simulink model "sampleModel56"  (Simulink 9.1)
settings: Solver=VariableStepAuto  StartTime=0.0  StopTime=10.0  RelTol=1e-3
undefined symbols (not defined in the file): DiscIntNeverNeededParam, Newton, Raphson
libraries: simulink x48
(part 2 of 2)

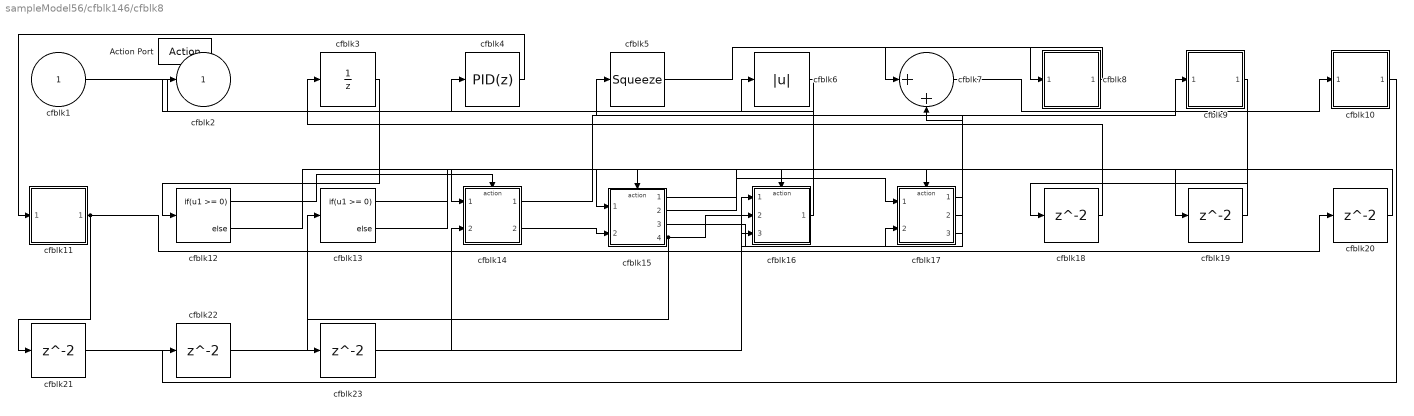
== system sampleModel56/cfblk146/cfblk8 ==
  cfblk1 : Inport
  Action Port : ActionPort  ActionType=then
  cfblk10 : Subsystem
  cfblk11 : Subsystem
  cfblk12 : If  IfExpression=u1 >= 0  SampleTime=1
  cfblk13 : If  IfExpression=u1 >= 0  SampleTime=1
  cfblk14 : Subsystem  TreatAsAtomicUnit=on
  cfblk15 : Subsystem  TreatAsAtomicUnit=on
  cfblk16 : Subsystem  TreatAsAtomicUnit=on
  cfblk17 : Subsystem  TreatAsAtomicUnit=on
  cfblk{18..23} (6 alike) : Delay
  cfblk3 : UnitDelay  SampleTime=-1
  cfblk4 : simulink/Continuous/PID Controller  Controller=PID  TimeDomain=Discrete-time  SampleTime=-1  IntegratorMethod=Forward Euler  FilterMethod=Forward Euler  Form=Parallel  UseFilter=on  ControllerParametersSource=internal  P=1  I=1  D=0  N=100  InitialConditionSource=internal  InitialConditionForIntegrator=0  InitialConditionForFilter=0  ExternalReset=none  LimitOutput=off  UpperSaturationLimit=inf  LowerSaturationLimit=-inf  LinearizeAsGain=off  AntiWindupMode=none  Kb=1  TrackingMode=off  Kt=1  PParamMin=[]  PParamMax=[]  IParamMin=[]  IParamMax=[]  DParamMin=[]  DParamMax=[]  NParamMin=[]  NParamMax=[]  KbParamMin=[]  KbParamMax=[]  KtParamMin=[]  KtParamMax=[]  POutMin=[]  POutMax=[]  IOutMin=[]  IOutMax=[]  DOutMin=[]  DOutMax=[]  NOutMin=[]  NOutMax=[]  KbOutMin=[]  KbOutMax=[]  KtOutMin=[]  KtOutMax=[]  IntegratorOutMin=[]  IntegratorOutMax=[]  FilterOutMin=[]  FilterOutMax=[]  SumOutMin=[]  SumOutMax=[]  SumI1OutMin=[]  SumI1OutMax=[]  SumI2OutMin=[]  SumI2OutMax=[]  SumI3OutMin=[]  SumI3OutMax=[]  SumDOutMin=[]  SumDOutMax=[]  SaturationOutMin=[]  SaturationOutMax=[]  IntegratorContinuousStateAttributes=''  IntegratorStateMustResolveToSignalObject=off  IntegratorRTWStateStorageClass=Auto  FilterContinuousStateAttributes=''  FilterStateMustResolveToSignalObject=off  FilterRTWStateStorageClass=Auto  DifferentiatorICPrevScaledInput=0  DifferentiatorOutMin=[]  DifferentiatorOutMax=[]  FilterDiffOutCoefMin=[]  FilterDiffOutCoefMax=[]  SumDenOutMin=[]  SumDenOutMax=[]  SumNumOutMin=[]  SumNumOutMax=[]  ReciprocalOutMin=[]  ReciprocalOutMax=[]  DivideOutMin=[]  DivideOutMax=[]  TunerSelectOption=Transfer Function Based (PID Tuner App)
  cfblk5 : Squeeze
  cfblk6 : Abs
  cfblk7 : Sum  Inputs=|++
  cfblk8 : Subsystem
  cfblk9 : Subsystem
  cfblk2 : Outport
  wires:
  cfblk1/1 -> cfblk6/1
  cfblk3/1 -> cfblk12/1
  cfblk4/1 -> cfblk11/1(cfblk1)
  cfblk6/1 -> cfblk2/1
  cfblk5/1 -> cfblk8/1(cfblk1)
  cfblk16/1(cfblk2) -> cfblk4/1
  cfblk11/1(cfblk2) -> cfblk20/1, cfblk21/1
  cfblk7/1 -> cfblk10/1(cfblk1)
  cfblk14/1(cfblk2) -> cfblk9/1(cfblk1)
  cfblk8/1(cfblk2) -> cfblk7/1
  cfblk14/2(cfblk12) -> cfblk15/2(cfblk12)
  cfblk17/1(cfblk2) -> cfblk16/1(cfblk1)
  cfblk17/2(cfblk16) -> cfblk5/1
  cfblk17/3(cfblk17) -> cfblk7/2
  cfblk15/2(cfblk13) -> cfblk17/1(cfblk1)
  cfblk15/3(cfblk14) -> cfblk17/2(cfblk15)
  cfblk15/4(cfblk15) -> cfblk16/2(cfblk15), cfblk23/1
  cfblk12/1 -> cfblk14/Action
  cfblk12/2 -> cfblk15/Action
  cfblk13/1 -> cfblk16/Action
  cfblk13/2 -> cfblk17/Action
  cfblk9/1(cfblk2) -> cfblk18/1
  cfblk18/1 -> cfblk3/1
  cfblk15/1(cfblk2) -> cfblk19/1
  cfblk19/1 -> cfblk14/1(cfblk1)
  cfblk20/1 -> cfblk15/1(cfblk1)
  cfblk21/1 -> cfblk16/3(cfblk16)
  cfblk10/1(cfblk2) -> cfblk22/1
  cfblk22/1 -> cfblk13/1
  cfblk23/1 -> cfblk14/2(cfblk11)

== system sampleModel56/cfblk146/cfblk9 ==
  cfblk1 : Inport
  Action Port : ActionPort  ActionType=else
  cfblk3 : UnitDelay  SampleTime=-1
  cfblk4 : Product  Inputs=*
  cfblk5 : Subsystem
  cfblk6 : Subsystem
  cfblk7 : Subsystem
  cfblk8 : Subsystem
  cfblk2 : Outport
  cfblk9 : Outport  Port=2
  wires:
  cfblk1/1 -> cfblk8/1(cfblk1)
  cfblk8/1(cfblk2) -> cfblk6/1(cfblk1)
  cfblk6/1(cfblk2) -> cfblk7/1(cfblk1)
  cfblk7/1(cfblk2) -> cfblk3/1, cfblk5/1(cfblk1)
  cfblk3/1 -> cfblk2/1
  cfblk5/1(cfblk2) -> cfblk4/1
  cfblk4/1 -> cfblk9/1

== system sampleModel56/cfblk147/cfblk10 ==
  cfblk1 : Inport
  cfblk2 : Outport
  wires:
  cfblk1/1 -> cfblk2/1

== system sampleModel56/cfblk147/cfblk11 ==
  cfblk1 : Inport
  cfblk2 : Outport
  wires:
  cfblk1/1 -> cfblk2/1

== system sampleModel56/cfblk147/cfblk12 ==
  cfblk1 : Inport
  cfblk2 : Outport
  wires:
  cfblk1/1 -> cfblk2/1

== system sampleModel56/cfblk147/cfblk13 ==
  cfblk1 : Inport
  cfblk2 : Outport
  wires:
  cfblk1/1 -> cfblk2/1

== system sampleModel56/cfblk147/cfblk14 ==
  cfblk1 : Inport
  cfblk2 : Outport
  wires:
  cfblk1/1 -> cfblk2/1

== system sampleModel56/cfblk148/cfblk10 ==
  cfblk1 : Inport
  cfblk2 : Outport
  wires:
  cfblk1/1 -> cfblk2/1

== system sampleModel56/cfblk148/cfblk11 ==
  cfblk1 : Inport
  cfblk2 : Outport
  wires:
  cfblk1/1 -> cfblk2/1

== system sampleModel56/cfblk148/cfblk12 ==
  cfblk1 : Inport
  cfblk2 : Outport
  wires:
  cfblk1/1 -> cfblk2/1

== system sampleModel56/cfblk148/cfblk13 ==
  cfblk1 : Inport
  cfblk2 : Outport
  wires:
  cfblk1/1 -> cfblk2/1

== system sampleModel56/cfblk148/cfblk9 ==
  cfblk1 : Inport
  cfblk2 : Outport
  wires:
  cfblk1/1 -> cfblk2/1

== system sampleModel56/cfblk149/cfblk10 ==
  cfblk1 : Inport
  cfblk2 : Outport
  wires:
  cfblk1/1 -> cfblk2/1

== system sampleModel56/cfblk149/cfblk11 ==
  cfblk1 : Inport
  cfblk2 : Outport
  wires:
  cfblk1/1 -> cfblk2/1

== system sampleModel56/cfblk149/cfblk9 ==
  cfblk1 : Inport
  cfblk2 : Outport
  wires:
  cfblk1/1 -> cfblk2/1

== system sampleModel56/cfblk150/cfblk6 ==
  cfblk1 : Inport
  cfblk2 : Outport
  wires:
  cfblk1/1 -> cfblk2/1

== system sampleModel56/cfblk150/cfblk7 ==
  cfblk1 : Inport
  cfblk2 : Outport
  wires:
  cfblk1/1 -> cfblk2/1

== system sampleModel56/cfblk152/cfblk11 ==
  cfblk1 : Inport
  Action Port : ActionPort  ActionType=then
  cfblk10 : Subsystem
  cfblk11 : Subsystem
  cfblk3 : DiscreteTransferFcn
  cfblk4 : UnitDelay  SampleTime=-1
  cfblk5 : DiscreteIntegrator  SampleTime=-1  ICPrevOutput=DiscIntNeverNeededParam  ICPrevScaledInput=DiscIntNeverNeededParam
  cfblk6 : Sqrt  SaturateOnIntegerOverflow=on
  cfblk7 : Gain  Gain=[470576292.236771]
  cfblk8 : Subsystem
  cfblk9 : Subsystem
  cfblk2 : Outport
  cfblk12 : Outport  Port=2
  cfblk13 : Outport  Port=3
  wires:
  cfblk7/1 -> cfblk4/1
  cfblk6/1 -> cfblk7/1
  cfblk1/1 -> cfblk10/1(cfblk1)
  cfblk4/1 -> cfblk5/1
  cfblk11/1(cfblk2) -> cfblk8/1(cfblk1), cfblk2/1
  cfblk8/1(cfblk2) -> cfblk3/1
  cfblk3/1 -> cfblk12/1
  cfblk9/1(cfblk2) -> cfblk11/1(cfblk1)
  cfblk5/1 -> cfblk13/1, cfblk9/1(cfblk1)
  cfblk10/1(cfblk2) -> cfblk6/1

== system sampleModel56/cfblk152/cfblk12 ==
  cfblk1 : Inport
  cfblk9 : Inport  Port=2
  cfblk10 : Inport  Port=3
  Action Port : ActionPort  ActionType=else
  cfblk3 : UnitDelay  SampleTime=-1
  cfblk4 : Abs
  cfblk5 : Bias  Bias=[477951449.519788]
  cfblk6 : Signum
  cfblk7 : Subsystem
  cfblk8 : Subsystem
  cfblk2 : Outport
  wires:
  cfblk5/1 -> cfblk2/1
  cfblk6/1 -> cfblk4/1
  cfblk9/1 -> cfblk3/1
  cfblk4/1 -> cfblk8/1(cfblk1)
  cfblk10/1 -> cfblk5/1
  cfblk1/1 -> cfblk6/1
  cfblk8/1(cfblk2) -> cfblk7/1(cfblk1)

== system sampleModel56/cfblk152/cfblk6 ==
  cfblk1 : Inport
  cfblk2 : Outport
  wires:
  cfblk1/1 -> cfblk2/1

== system sampleModel56/cfblk152/cfblk7 ==
  cfblk1 : Inport
  cfblk2 : Outport
  wires:
  cfblk1/1 -> cfblk2/1

== system sampleModel56/cfblk152/cfblk8 ==
  cfblk1 : Inport
  cfblk2 : Outport
  wires:
  cfblk1/1 -> cfblk2/1

== system sampleModel56/cfblk153/cfblk11 ==
  cfblk1 : Inport
  cfblk2 : Outport
  wires:
  cfblk1/1 -> cfblk2/1

== system sampleModel56/cfblk153/cfblk12 ==
  cfblk1 : Inport
  cfblk2 : Outport
  wires:
  cfblk1/1 -> cfblk2/1

== system sampleModel56/cfblk154/cfblk11 ==
  cfblk1 : Inport
  cfblk2 : Outport
  wires:
  cfblk1/1 -> cfblk2/1

== system sampleModel56/cfblk154/cfblk12 ==
  cfblk1 : Inport
  cfblk2 : Outport
  wires:
  cfblk1/1 -> cfblk2/1

== system sampleModel56/cfblk154/cfblk13 ==
  cfblk1 : Inport
  cfblk2 : Outport
  wires:
  cfblk1/1 -> cfblk2/1

== system sampleModel56/cfblk154/cfblk14 ==
  cfblk1 : Inport
  cfblk2 : Outport
  wires:
  cfblk1/1 -> cfblk2/1

== system sampleModel56/cfblk155/cfblk10 ==
  cfblk1 : Inport
  cfblk2 : Outport
  wires:
  cfblk1/1 -> cfblk2/1

== system sampleModel56/cfblk155/cfblk7 ==
  cfblk1 : Inport
  cfblk2 : Outport
  wires:
  cfblk1/1 -> cfblk2/1

== system sampleModel56/cfblk155/cfblk8 ==
  cfblk1 : Inport
  cfblk2 : Outport
  wires:
  cfblk1/1 -> cfblk2/1

== system sampleModel56/cfblk155/cfblk9 ==
  cfblk1 : Inport
  cfblk2 : Outport
  wires:
  cfblk1/1 -> cfblk2/1

== system sampleModel56/cfblk156/cfblk10 ==
  cfblk1 : Inport
  cfblk2 : Outport
  wires:
  cfblk1/1 -> cfblk2/1

== system sampleModel56/cfblk156/cfblk11 ==
  cfblk1 : Inport
  cfblk2 : Outport
  wires:
  cfblk1/1 -> cfblk2/1

== system sampleModel56/cfblk156/cfblk12 ==
  cfblk1 : Inport
  cfblk2 : Outport
  wires:
  cfblk1/1 -> cfblk2/1

== system sampleModel56/cfblk156/cfblk9 ==
  cfblk1 : Inport
  cfblk2 : Outport
  wires:
  cfblk1/1 -> cfblk2/1

== system sampleModel56/cfblk157/cfblk7 ==
  cfblk1 : Inport
  cfblk2 : Outport
  wires:
  cfblk1/1 -> cfblk2/1

== system sampleModel56/cfblk157/cfblk8 ==
  cfblk1 : Inport
  cfblk2 : Outport
  wires:
  cfblk1/1 -> cfblk2/1

== system sampleModel56/cfblk158/cfblk10 ==
  cfblk1 : Inport
  cfblk2 : Outport
  wires:
  cfblk1/1 -> cfblk2/1

== system sampleModel56/cfblk158/cfblk11 ==
  cfblk1 : Inport
  cfblk2 : Outport
  wires:
  cfblk1/1 -> cfblk2/1

== system sampleModel56/cfblk158/cfblk12 ==
  cfblk1 : Inport
  cfblk2 : Outport
  wires:
  cfblk1/1 -> cfblk2/1

== system sampleModel56/cfblk158/cfblk13 ==
  cfblk1 : Inport
  cfblk2 : Outport
  wires:
  cfblk1/1 -> cfblk2/1

== system sampleModel56/cfblk158/cfblk14 ==
  cfblk1 : Inport
  cfblk2 : Outport
  wires:
  cfblk1/1 -> cfblk2/1

== system sampleModel56/cfblk158/cfblk15 ==
  cfblk1 : Inport
  cfblk2 : Outport
  wires:
  cfblk1/1 -> cfblk2/1

== system sampleModel56/cfblk158/cfblk8 ==
  cfblk1 : Inport
  cfblk2 : Outport
  wires:
  cfblk1/1 -> cfblk2/1

== system sampleModel56/cfblk158/cfblk9 ==
  cfblk1 : Inport
  cfblk2 : Outport
  wires:
  cfblk1/1 -> cfblk2/1

== system sampleModel56/cfblk146/cfblk8/cfblk10 ==
  cfblk1 : Inport
  cfblk2 : Outport
  wires:
  cfblk1/1 -> cfblk2/1

== system sampleModel56/cfblk146/cfblk8/cfblk11 ==
  cfblk1 : Inport
  cfblk2 : Outport
  wires:
  cfblk1/1 -> cfblk2/1

== system sampleModel56/cfblk146/cfblk8/cfblk14 ==
  cfblk1 : Inport
  cfblk11 : Inport  Port=2
  Action Port : ActionPort  ActionType=then
  cfblk10 : Subsystem
  cfblk13 : Delay
  cfblk14 : Delay
  cfblk3 : DiscreteTransferFcn
  cfblk4 : Delay  ShowEnablePort=on
      settings: InputPortMap=u0,e6
  cfblk5 : Sqrt  SaturateOnIntegerOverflow=on
  cfblk6 : Reshape
  cfblk7 : DotProduct  InputSameDT=on  OutDataTypeStr=Inherit: Inherit via internal rule
  cfblk8 : Product  Inputs=*
  cfblk9 : Subsystem
  cfblk2 : Outport
  cfblk12 : Outport  Port=2
  wires:
  cfblk4/1 -> cfblk9/1(cfblk1), cfblk7/2, cfblk6/1
  cfblk11/1 -> cfblk12/1
  cfblk3/1 -> cfblk10/1(cfblk1)
  cfblk6/1 -> cfblk5/1
  cfblk1/1 -> cfblk8/1
  cfblk5/1 -> cfblk7/1
  cfblk8/1 -> cfblk4/2
  cfblk7/1 -> cfblk2/1
  cfblk9/1(cfblk2) -> cfblk13/1
  cfblk13/1 -> cfblk4/1
  cfblk10/1(cfblk2) -> cfblk14/1
  cfblk14/1 -> cfblk3/1

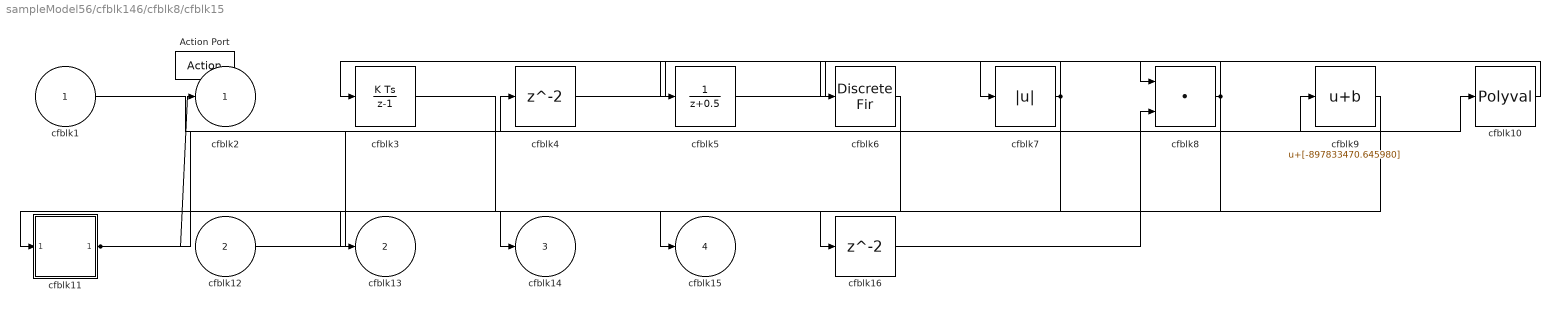
== system sampleModel56/cfblk146/cfblk8/cfblk15 ==
  cfblk1 : Inport
  cfblk12 : Inport  Port=2
  Action Port : ActionPort  ActionType=else
  cfblk10 : Polyval  Coefs=[ +2.081618890e-019, -1.441693666e-014, +4.719686976e-010, -8.536869453e-006, +1.621573104e-001, -8.087801117e+001 ]
  cfblk11 : Subsystem
  cfblk16 : Delay
  cfblk3 : DiscreteIntegrator  SampleTime=-1  ICPrevOutput=DiscIntNeverNeededParam  ICPrevScaledInput=DiscIntNeverNeededParam
  cfblk4 : Delay
  cfblk5 : DiscreteTransferFcn
  cfblk6 : DiscreteFir
  cfblk7 : Abs
  cfblk8 : DotProduct  InputSameDT=on  OutDataTypeStr=Inherit: Inherit via internal rule
  cfblk9 : Bias  Bias=[-897833470.645980]
  cfblk2 : Outport
  cfblk13 : Outport  Port=2
  cfblk14 : Outport  Port=3
  cfblk15 : Outport  Port=4
  wires:
  cfblk9/1 -> cfblk14/1
  cfblk12/1 -> cfblk9/1
  cfblk10/1 -> cfblk3/1
  cfblk4/1 -> cfblk8/1
  cfblk1/1 -> cfblk4/1
  cfblk6/1 -> cfblk15/1
  cfblk5/1 -> cfblk7/1
  cfblk7/1 -> cfblk6/1, cfblk13/1
  cfblk8/1 -> cfblk5/1, cfblk11/1(cfblk1)
  cfblk11/1(cfblk2) -> cfblk2/1, cfblk10/1
  cfblk3/1 -> cfblk16/1
  cfblk16/1 -> cfblk8/2

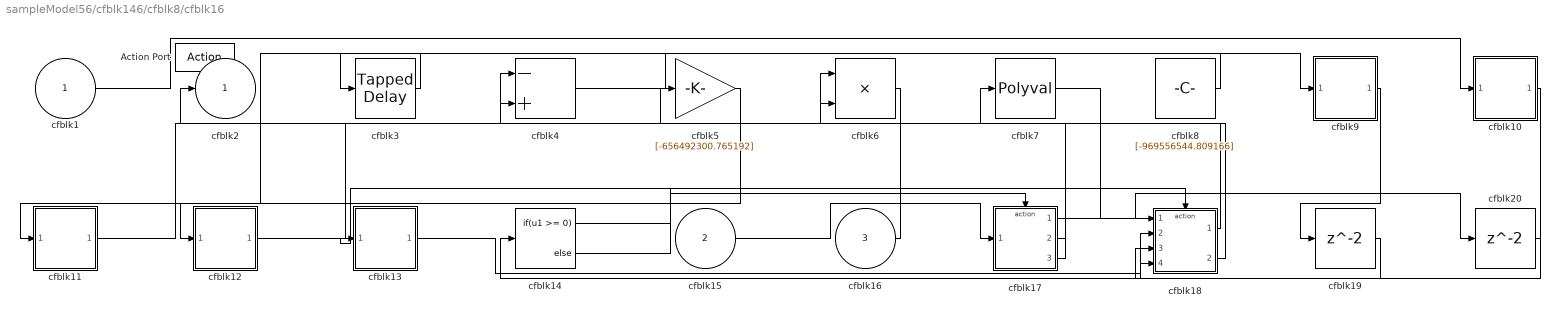
== system sampleModel56/cfblk146/cfblk8/cfblk16 ==
  cfblk1 : Inport
  cfblk15 : Inport  Port=2
  cfblk16 : Inport  Port=3
  Action Port : ActionPort  ActionType=then
  cfblk10 : Subsystem
  cfblk11 : Subsystem
  cfblk12 : Subsystem
  cfblk13 : Subsystem
  cfblk14 : If  IfExpression=u1 >= 0  SampleTime=1
  cfblk17 : Subsystem  TreatAsAtomicUnit=on
  cfblk18 : Subsystem  TreatAsAtomicUnit=on
  cfblk19 : Delay
  cfblk20 : Delay
  cfblk3 : simulink/Discrete/Tapped Delay  vinit=0.0  samptime=-1  NumDelays=1  DelayOrder=Oldest  includeCurrent=off
  cfblk4 : Sum  Inputs=-+
  cfblk5 : Gain  Gain=[-656492300.765192]
  cfblk6 : Product  Inputs=**
  cfblk7 : Polyval  Coefs=[ +2.081618890e-019, -1.441693666e-014, +4.719686976e-010, -8.536869453e-006, +1.621573104e-001, -8.087801117e+001 ]
  cfblk8 : Constant  Value=[-969556544.809166]  SampleTime=1
  cfblk9 : Subsystem
  cfblk2 : Outport
  wires:
  cfblk7/1 -> cfblk18/1(cfblk1)
  cfblk10/1(cfblk2) -> cfblk18/2(cfblk8)
  cfblk12/1(cfblk2) -> cfblk4/1
  cfblk6/1 -> cfblk13/1(cfblk1)
  cfblk3/1 -> cfblk12/1(cfblk1)
  cfblk15/1 -> cfblk17/1(cfblk1)
  cfblk8/1 -> cfblk3/1
  cfblk1/1 -> cfblk10/1(cfblk1)
  cfblk4/1 -> cfblk9/1(cfblk1)
  cfblk18/1(cfblk2) -> cfblk5/1
  cfblk16/1 -> cfblk6/1
  cfblk11/1(cfblk2) -> cfblk4/2
  cfblk17/2(cfblk12) -> cfblk6/2
  cfblk18/2(cfblk11) -> cfblk2/1
  cfblk13/1(cfblk2) -> cfblk18/4(cfblk10)
  cfblk17/3(cfblk13) -> cfblk7/1
  cfblk5/1 -> cfblk11/1(cfblk1)
  cfblk14/1 -> cfblk17/Action
  cfblk14/2 -> cfblk18/Action
  cfblk9/1(cfblk2) -> cfblk19/1
  cfblk19/1 -> cfblk18/3(cfblk9)
  cfblk17/1(cfblk2) -> cfblk20/1
  cfblk20/1 -> cfblk14/1

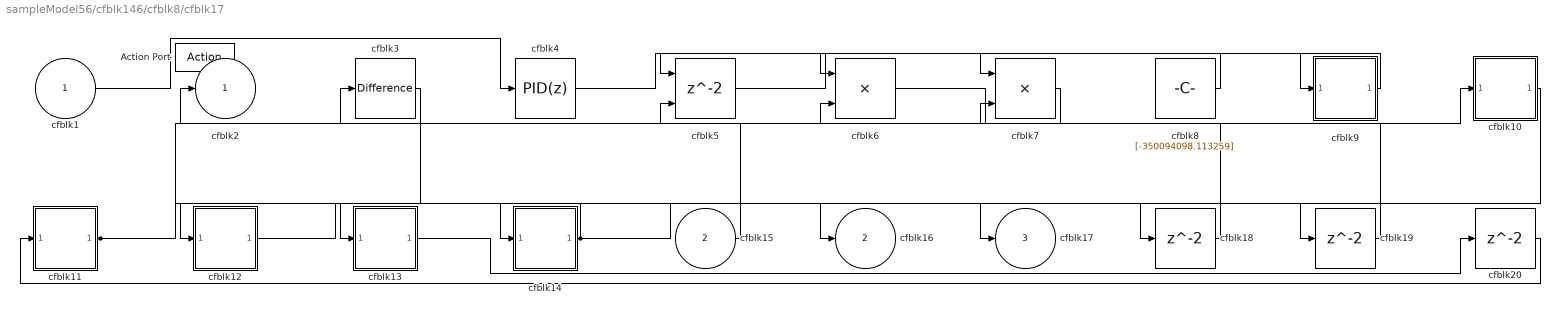
== system sampleModel56/cfblk146/cfblk8/cfblk17 ==
  cfblk1 : Inport
  cfblk15 : Inport  Port=2
  Action Port : ActionPort  ActionType=else
  cfblk10 : Subsystem
  cfblk11 : Subsystem
  cfblk12 : Subsystem
  cfblk13 : Subsystem
  cfblk14 : Subsystem
  cfblk18 : Delay
  cfblk19 : Delay
  cfblk20 : Delay
  cfblk3 : simulink/Discrete/Difference  ICPrevInput=0.0  OutMin=[]  OutMax=[]  OutDataTypeStr=Inherit: Inherit via back propagation  OutDataType=fixdt(1, 16)  OutScaling=2^-10  DoSatur=off
  cfblk4 : simulink/Continuous/PID Controller  Controller=PID  TimeDomain=Discrete-time  SampleTime=-1  IntegratorMethod=Forward Euler  FilterMethod=Forward Euler  Form=Parallel  UseFilter=on  ControllerParametersSource=internal  P=1  I=1  D=0  N=100  InitialConditionSource=internal  InitialConditionForIntegrator=0  InitialConditionForFilter=0  ExternalReset=none  LimitOutput=off  UpperSaturationLimit=inf  LowerSaturationLimit=-inf  LinearizeAsGain=off  AntiWindupMode=none  Kb=1  TrackingMode=off  Kt=1  PParamMin=[]  PParamMax=[]  IParamMin=[]  IParamMax=[]  DParamMin=[]  DParamMax=[]  NParamMin=[]  NParamMax=[]  KbParamMin=[]  KbParamMax=[]  KtParamMin=[]  KtParamMax=[]  POutMin=[]  POutMax=[]  IOutMin=[]  IOutMax=[]  DOutMin=[]  DOutMax=[]  NOutMin=[]  NOutMax=[]  KbOutMin=[]  KbOutMax=[]  KtOutMin=[]  KtOutMax=[]  IntegratorOutMin=[]  IntegratorOutMax=[]  FilterOutMin=[]  FilterOutMax=[]  SumOutMin=[]  SumOutMax=[]  SumI1OutMin=[]  SumI1OutMax=[]  SumI2OutMin=[]  SumI2OutMax=[]  SumI3OutMin=[]  SumI3OutMax=[]  SumDOutMin=[]  SumDOutMax=[]  SaturationOutMin=[]  SaturationOutMax=[]  IntegratorContinuousStateAttributes=''  IntegratorStateMustResolveToSignalObject=off  IntegratorRTWStateStorageClass=Auto  FilterContinuousStateAttributes=''  FilterStateMustResolveToSignalObject=off  FilterRTWStateStorageClass=Auto  DifferentiatorICPrevScaledInput=0  DifferentiatorOutMin=[]  DifferentiatorOutMax=[]  FilterDiffOutCoefMin=[]  FilterDiffOutCoefMax=[]  SumDenOutMin=[]  SumDenOutMax=[]  SumNumOutMin=[]  SumNumOutMax=[]  ReciprocalOutMin=[]  ReciprocalOutMax=[]  DivideOutMin=[]  DivideOutMax=[]  TunerSelectOption=Transfer Function Based (PID Tuner App)
  cfblk5 : Delay  ShowEnablePort=on
      settings: InputPortMap=u0,e6
  cfblk6 : Product  Inputs=**
  cfblk7 : Product
  cfblk8 : Constant  Value=[-350094098.113259]  SampleTime=1
  cfblk9 : Subsystem
  cfblk2 : Outport
  cfblk16 : Outport  Port=2
  cfblk17 : Outport  Port=3
  wires:
  cfblk15/1 -> cfblk2/1
  cfblk8/1 -> cfblk5/1
  cfblk3/1 -> cfblk12/1(cfblk1)
  cfblk7/1 -> cfblk5/2
  cfblk1/1 -> cfblk4/1
  cfblk5/1 -> cfblk9/1(cfblk1)
  cfblk14/1(cfblk2) -> cfblk13/1(cfblk1), cfblk17/1
  cfblk4/1 -> cfblk7/1
  cfblk6/1 -> cfblk10/1(cfblk1)
  cfblk11/1(cfblk2) -> cfblk7/2, cfblk16/1, cfblk14/1(cfblk1)
  cfblk9/1(cfblk2) -> cfblk6/1
  cfblk10/1(cfblk2) -> cfblk18/1
  cfblk18/1 -> cfblk6/2
  cfblk12/1(cfblk2) -> cfblk19/1
  cfblk19/1 -> cfblk3/1
  cfblk13/1(cfblk2) -> cfblk20/1
  cfblk20/1 -> cfblk11/1(cfblk1)

== system sampleModel56/cfblk146/cfblk8/cfblk8 ==
  cfblk1 : Inport
  cfblk2 : Outport
  wires:
  cfblk1/1 -> cfblk2/1

== system sampleModel56/cfblk146/cfblk8/cfblk9 ==
  cfblk1 : Inport
  cfblk2 : Outport
  wires:
  cfblk1/1 -> cfblk2/1

== system sampleModel56/cfblk146/cfblk9/cfblk5 ==
  cfblk1 : Inport
  cfblk2 : Outport
  wires:
  cfblk1/1 -> cfblk2/1

== system sampleModel56/cfblk146/cfblk9/cfblk6 ==
  cfblk1 : Inport
  cfblk2 : Outport
  wires:
  cfblk1/1 -> cfblk2/1

== system sampleModel56/cfblk146/cfblk9/cfblk7 ==
  cfblk1 : Inport
  cfblk2 : Outport
  wires:
  cfblk1/1 -> cfblk2/1

== system sampleModel56/cfblk146/cfblk9/cfblk8 ==
  cfblk1 : Inport
  cfblk2 : Outport
  wires:
  cfblk1/1 -> cfblk2/1

== system sampleModel56/cfblk152/cfblk11/cfblk10 ==
  cfblk1 : Inport
  cfblk2 : Outport
  wires:
  cfblk1/1 -> cfblk2/1

== system sampleModel56/cfblk152/cfblk11/cfblk11 ==
  cfblk1 : Inport
  cfblk2 : Outport
  wires:
  cfblk1/1 -> cfblk2/1

== system sampleModel56/cfblk152/cfblk11/cfblk8 ==
  cfblk1 : Inport
  cfblk2 : Outport
  wires:
  cfblk1/1 -> cfblk2/1

== system sampleModel56/cfblk152/cfblk11/cfblk9 ==
  cfblk1 : Inport
  cfblk2 : Outport
  wires:
  cfblk1/1 -> cfblk2/1

== system sampleModel56/cfblk152/cfblk12/cfblk7 ==
  cfblk1 : Inport
  cfblk2 : Outport
  wires:
  cfblk1/1 -> cfblk2/1

== system sampleModel56/cfblk152/cfblk12/cfblk8 ==
  cfblk1 : Inport
  cfblk2 : Outport
  wires:
  cfblk1/1 -> cfblk2/1

== system sampleModel56/cfblk146/cfblk8/cfblk14/cfblk10 ==
  cfblk1 : Inport
  cfblk2 : Outport
  wires:
  cfblk1/1 -> cfblk2/1

== system sampleModel56/cfblk146/cfblk8/cfblk14/cfblk9 ==
  cfblk1 : Inport
  cfblk2 : Outport
  wires:
  cfblk1/1 -> cfblk2/1

== system sampleModel56/cfblk146/cfblk8/cfblk15/cfblk11 ==
  cfblk1 : Inport
  cfblk2 : Outport
  wires:
  cfblk1/1 -> cfblk2/1

== system sampleModel56/cfblk146/cfblk8/cfblk16/cfblk10 ==
  cfblk1 : Inport
  cfblk2 : Outport
  wires:
  cfblk1/1 -> cfblk2/1

== system sampleModel56/cfblk146/cfblk8/cfblk16/cfblk11 ==
  cfblk1 : Inport
  cfblk2 : Outport
  wires:
  cfblk1/1 -> cfblk2/1

== system sampleModel56/cfblk146/cfblk8/cfblk16/cfblk12 ==
  cfblk1 : Inport
  cfblk2 : Outport
  wires:
  cfblk1/1 -> cfblk2/1

== system sampleModel56/cfblk146/cfblk8/cfblk16/cfblk13 ==
  cfblk1 : Inport
  cfblk2 : Outport
  wires:
  cfblk1/1 -> cfblk2/1

== system sampleModel56/cfblk146/cfblk8/cfblk16/cfblk17 ==
  cfblk1 : Inport
  Action Port : ActionPort  ActionType=then
  cfblk10 : ComplexToRealImag
  cfblk11 : Trigonometry
  cfblk14 : Delay
  cfblk15 : Delay
  cfblk3 : simulink/Discrete/Transfer Fcn Real Zero  ZeroZ=0.75  ICPrevInput=0.0  DoSatur=off
      settings: SourceProductName=Simulink  SourceProductBaseCode=SL
  cfblk4 : DotProduct  InputSameDT=on  OutDataTypeStr=Inherit: Inherit via internal rule
  cfblk5 : Assignment  DiagnosticForDimensions=Warning  IndexOptions=Index vector (dialog)  Indices=1  OutputSizes=1
  cfblk6 : Product  Inputs=**
  cfblk7 : Sum  Inputs=+-
  cfblk8 : Sqrt  SaturateOnIntegerOverflow=on
  cfblk9 : Sin  TimeSource=Use external signal  SampleTime=0
  cfblk2 : Outport
  cfblk12 : Outport  Port=2
  cfblk13 : Outport  Port=3
  wires:
  cfblk11/1 -> cfblk6/1, cfblk8/1, cfblk12/1
  cfblk6/1 -> cfblk5/1
  cfblk3/1 -> cfblk4/1, cfblk7/2
  cfblk9/1 -> cfblk5/2, cfblk14/1
  cfblk10/1 -> cfblk13/1
  cfblk4/1 -> cfblk7/1, cfblk11/1
  cfblk7/1 -> cfblk9/1
  cfblk5/1 -> cfblk10/1
  cfblk10/2 -> cfblk2/1
  cfblk1/1 -> cfblk6/2
  cfblk14/1 -> cfblk4/2
  cfblk8/1 -> cfblk15/1
  cfblk15/1 -> cfblk3/1

== system sampleModel56/cfblk146/cfblk8/cfblk16/cfblk18 ==
  cfblk1 : Inport
  cfblk8 : Inport  Port=2
  cfblk9 : Inport  Port=3
  cfblk10 : Inport  Port=4
  Action Port : ActionPort  ActionType=else
  cfblk3 : PermuteDimensions
  cfblk4 : MinMax  Function=max
  cfblk5 : Sum  Inputs=+-
  cfblk6 : Constant  Value=[-697074411.304134]  SampleTime=1
  cfblk7 : Constant  Value=[-350148001.758244]  SampleTime=1
  cfblk2 : Outport
  cfblk11 : Outport  Port=2
  wires:
  cfblk1/1 -> cfblk3/1
  cfblk3/1 -> cfblk2/1
  cfblk6/1 -> cfblk5/1
  cfblk5/1 -> cfblk11/1
  cfblk7/1 -> cfblk5/2
  cfblk9/1 -> cfblk4/1

== system sampleModel56/cfblk146/cfblk8/cfblk16/cfblk9 ==
  cfblk1 : Inport
  cfblk2 : Outport
  wires:
  cfblk1/1 -> cfblk2/1

== system sampleModel56/cfblk146/cfblk8/cfblk17/cfblk10 ==
  cfblk1 : Inport
  cfblk2 : Outport
  wires:
  cfblk1/1 -> cfblk2/1

== system sampleModel56/cfblk146/cfblk8/cfblk17/cfblk11 ==
  cfblk1 : Inport
  cfblk2 : Outport
  wires:
  cfblk1/1 -> cfblk2/1

== system sampleModel56/cfblk146/cfblk8/cfblk17/cfblk12 ==
  cfblk1 : Inport
  cfblk2 : Outport
  wires:
  cfblk1/1 -> cfblk2/1

== system sampleModel56/cfblk146/cfblk8/cfblk17/cfblk13 ==
  cfblk1 : Inport
  cfblk2 : Outport
  wires:
  cfblk1/1 -> cfblk2/1

== system sampleModel56/cfblk146/cfblk8/cfblk17/cfblk14 ==
  cfblk1 : Inport
  cfblk2 : Outport
  wires:
  cfblk1/1 -> cfblk2/1

== system sampleModel56/cfblk146/cfblk8/cfblk17/cfblk9 ==
  cfblk1 : Inport
  cfblk2 : Outport
  wires:
  cfblk1/1 -> cfblk2/1
